simulink library "dec"  (Simulink 8.1)
settings: Solver=ode1  StartTime=0.0  StopTime=Inf  FixedStep=0.001  RelTol=1e-3
PostLoadFcn:
  | , if any(exist('dsrtsu_mdlpostloadfcn', 'file') == [2, 3, 6]), try dsrtsu_mdlpostloadfcn('Execute', bdroot); catch fprintf('Error in PostLoadFcn (dsrtsu_mdlpostloadfcn) for model "%s":\n %s\n', bdroot, lasterr); end, end,
undefined symbols (not defined in the file or in its folder): ZERO_FLOAT
libraries: drc x1, drf x1
settings Model: DSRTSU_INTERNAL_RTI_VER=450  DSRTSU_INTERNAL_RTI_TYPE=rti1401  RTICANMMDATA=struct('GeneralSetupData',struct('modelroot','D:\ELN150201_TAIWAN\trunk\AdasDragon\software\sw_development\arch\app\acc','generalsettings',struct('filesettings',struct('destfolder',struct('Name','RTICANMM_FILES','Check',1),'buildfolder',struct('Name','.','Check',1),'AbsDestfolder',struct('Name','D:\ELN150201_TAIWAN\trunk\AdasDragon\software\sw_development\arch\app\acc\RTICANMM_FILES'),'AbsBuildfolder',struct('Name','D:\ELN150201_TAIWAN\trunk\AdasDragon\software\sw_development\arch\app\acc'))),'options',struct('addpaths',1,'rmpaths',1,'addtrcexclusion',logical(1),'cannavigator',struct('checkmonitoring',0),'show_usrtrc',0,'use_usrtrc',0),'advanced',struct('options',[1 1 1 1 1 1 1 1 1 1 1 1 1 1 1 1 1 1 1 1 1 1 1 1 1 1 1 1 1 1 1 1 1 1 1 1 1 1 1 1 1 1 1 1 1 1 1 1 1 1 1 1 1 1 1 1 1 1 1 1 1 1 1 1 1 1 1 1 1 1 1 1 1 1 1 1 1 1 1 1 1 1 1 1 1 1 1 1 1 1 1 1 1 1 1 1 1 1 1 1]),'MPSetup',{{}},'modelname','dec','block','dec'))  DSRTSU_INTERNAL_RTIFPGA=40  Creator=AT015411  LastModifiedBy=AT015555

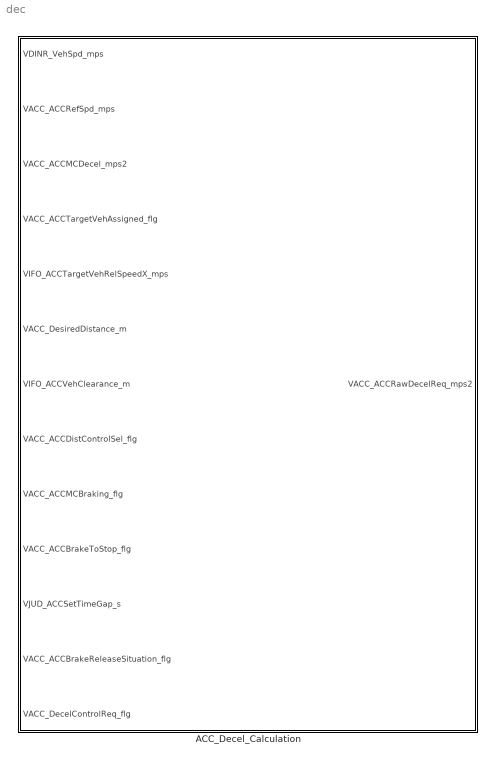
== system dec ==
  ACC_Decel_Calculation : Subsystem

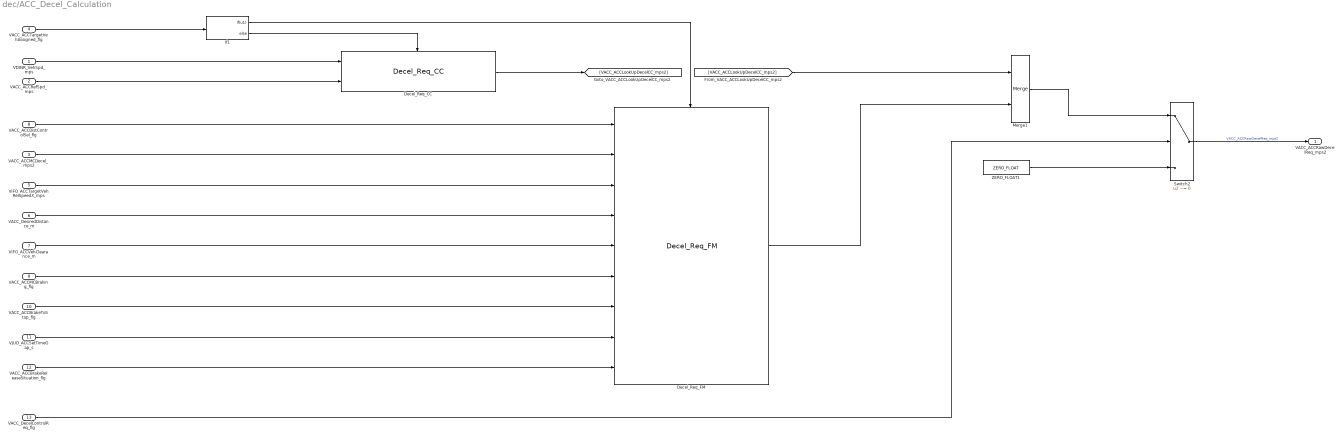
== system dec/ACC_Decel_Calculation ==
  VDINR_VehSpd_mps : Inport
  VACC_ACCRefSpd_mps : Inport  Port=2
  VACC_ACCMCDecel_mps2 : Inport  Port=3
  VACC_ACCTargetVehAssigned_flg : Inport  Port=4
  VIFO_ACCTargetVehRelSpeedX_mps : Inport  Port=5
  VACC_DesiredDistance_m : Inport  Port=6
  VIFO_ACCVehClearance_m : Inport  Port=7
  VACC_ACCDistControlSel_flg : Inport  Port=8
  VACC_ACCMCBraking_flg : Inport  Port=9
  VACC_ACCBrakeToStop_flg : Inport  Port=10
  VJUD_ACCSetTimeGap_s : Inport  Port=11
  VACC_ACCBrakeReleaseSituation_flg : Inport  Port=12
  VACC_DecelControlReq_flg : Inport  Port=13
  Decel_Req_CC : drc/Decel_Req_CC
  Decel_Req_FM : drf/Decel_Req_FM
  If1 : If  IfExpression=u1
  Merge1 : Merge
  Switch2 : Switch  Criteria=u2 ~= 0
  ZERO_FLOAT1 : Constant  Value=ZERO_FLOAT  OutDataTypeStr=single
  VACC_ACCRawDecelReq_mps2 : Outport
  wires:
  Switch2/1 -> VACC_ACCRawDecelReq_mps2/1  "VACC_ACCRawDecelReq_mps2"
  ZERO_FLOAT1/1 -> Switch2/3
  VACC_DecelControlReq_flg/1 -> Switch2/2
  VDINR_VehSpd_mps/1 -> Decel_Req_CC/1
  VACC_ACCRefSpd_mps/1 -> Decel_Req_CC/2
  VACC_ACCTargetVehAssigned_flg/1 -> If1/1
  If1/1 -> Decel_Req_FM/Action
  If1/2 -> Decel_Req_CC/Action
  Decel_Req_FM/1 -> Merge1/2
  [VACC_ACCLookUpDecelCC_mps2] -> Merge1/1
  Decel_Req_CC/1 -> [VACC_ACCLookUpDecelCC_mps2]
  Merge1/1 -> Switch2/1
  VACC_ACCDistControlSel_flg/1 -> Decel_Req_FM/1
  VACC_DesiredDistance_m/1 -> Decel_Req_FM/4
  VIFO_ACCTargetVehRelSpeedX_mps/1 -> Decel_Req_FM/3
  VIFO_ACCVehClearance_m/1 -> Decel_Req_FM/5
  VACC_ACCMCDecel_mps2/1 -> Decel_Req_FM/2
  VACC_ACCMCBraking_flg/1 -> Decel_Req_FM/6
  VACC_ACCBrakeToStop_flg/1 -> Decel_Req_FM/7
  VJUD_ACCSetTimeGap_s/1 -> Decel_Req_FM/8
  VACC_ACCBrakeReleaseSituation_flg/1 -> Decel_Req_FM/9
